simulink model "unit_test"  (R2019a)
settings: Solver=VariableStepAuto  StartTime=0.0  StopTime=inf  RelTol=1e-3
settings Model: Creator=anton  LastModifiedBy=anton

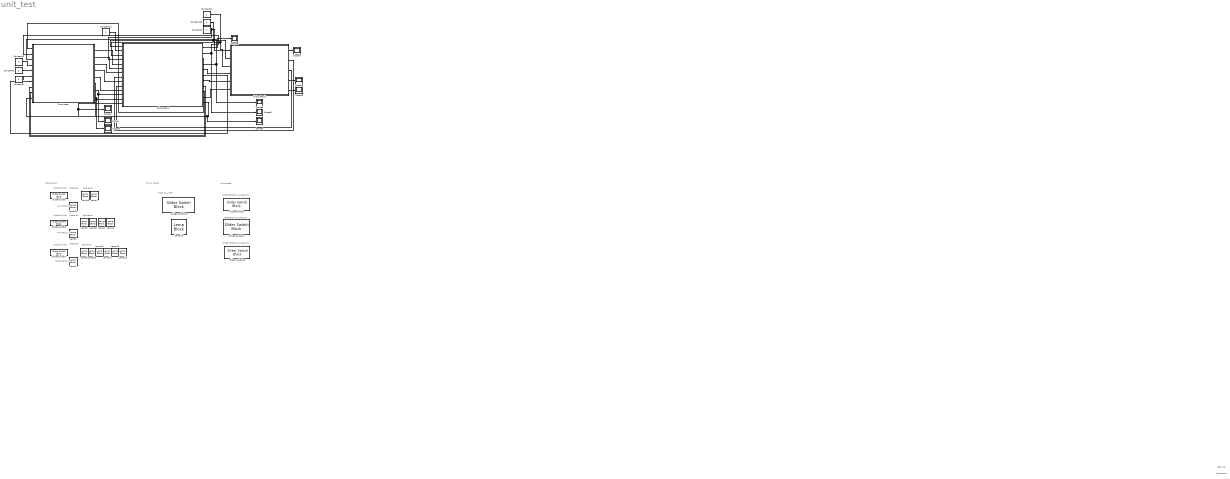
== system unit_test ==
  note: OPERATORE AVAILABILITY
  note: UTENSILE AVAILABILITY
  note: WORKSPACE AVAILABILITY
  note: Workspace
  note: TURN ON / OFF
  note: Pick & Place
  note: Place Pezzo 3
  note: Pick Pezzo 2
  note: Pick Pezzo1
  note: Capienza
  note: Capienza
  note: Capienza
  note: Disponibilità
  note: Scatola3
  note: Scatola2
  note: Scatola1
  note: Warehouse
  note: Operatore
  note: Utensile
  note: Disponibilità
  note: Disponibilità
  Constant{1..4,10..12} (7 alike) : Constant
  Lamp{1..16} (16 alike) : LampBlock
  Scope{,1..9} (10 alike) : Scope
  Slider Switch{,5,7,9,11..13} (7 alike) : SliderSwitchBlock
      settings: Values={{'Off', 'On'}, [0 1]}
  Subsystem : Subsystem
      mask Display: image('F:\MEGAsync\libri\Master\04_Model_Based\Esame\Model-Based-Master\Pick&Place\Immagini\000228601_FR_scatola-cartone-avana-imballi.jpg');
  Subsystem1 : Subsystem
      mask Display: image('967_z_pick_and_place.210.jpg');
  Subsystem2 : Subsystem
      mask Display: image('F:\MEGAsync\libri\Master\04_Model_Based\Esame\Model-Based-Master\Pick&Place\Immagini\download.jpg');
  wires:
  Constant2/1 -> Subsystem2/1(In1), Subsystem1/4(In4)
  Constant12/1 -> Subsystem1/1(In1), Subsystem2/2(In2)
  Constant11/1 -> Subsystem2/3(In3), Subsystem1/3(In3)
  Constant1/1 -> Subsystem/4(In4)
  Constant3/1 -> Subsystem/5(In5)
  Constant4/1 -> Subsystem/6(In6)
  Subsystem2/1(Out1) -> Scope7/1
  Subsystem2/4(Out4) -> Scope8/1
  Subsystem2/5(Out5) -> Scope9/1
  Subsystem/7(Out7) -> Scope/1, Subsystem1/12(In12)
  Subsystem/6(Out6) -> Subsystem1/14(In14), Scope1/1
  Subsystem/8(Out8) -> Scope2/1, Subsystem1/13(In13)
  Subsystem1/4(Out4) -> Scope5/1, Subsystem/3(In3)
  Subsystem1/2(Out2) -> Scope3/1, Subsystem/2(In2)
  Subsystem1/11(Out11) -> Subsystem/10(In10), Scope4/1
  Constant10/1 -> Subsystem1/2(In2)
  Subsystem/1(Out1) -> Subsystem1/5(In5)
  Subsystem/2(Out2) -> Subsystem1/6(In6)
  Subsystem/3(Out3) -> Subsystem1/7(In7)
  Subsystem2/2(Out2) -> Subsystem1/8(In8)
  Subsystem/4(Out4) -> Subsystem1/9(In9)
  Subsystem2/3(Out3) -> Subsystem1/10(In10)
  Subsystem/5(Out5) -> Subsystem1/11(In11)
  Subsystem1/1(Out1) -> Scope6/1
  Subsystem1/3(Out3) -> Subsystem/1(In1)
  Subsystem1/5(Out5) -> Subsystem2/4(In4)
  Subsystem1/6(Out6) -> Subsystem/7(In7)
  Subsystem1/7(Out7) -> Subsystem2/5(In5)
  Subsystem1/8(Out8) -> Subsystem/8(In8)
  Subsystem1/9(Out9) -> Subsystem/9(In9)
  Subsystem1/10(Out10) -> Subsystem2/6(In6)

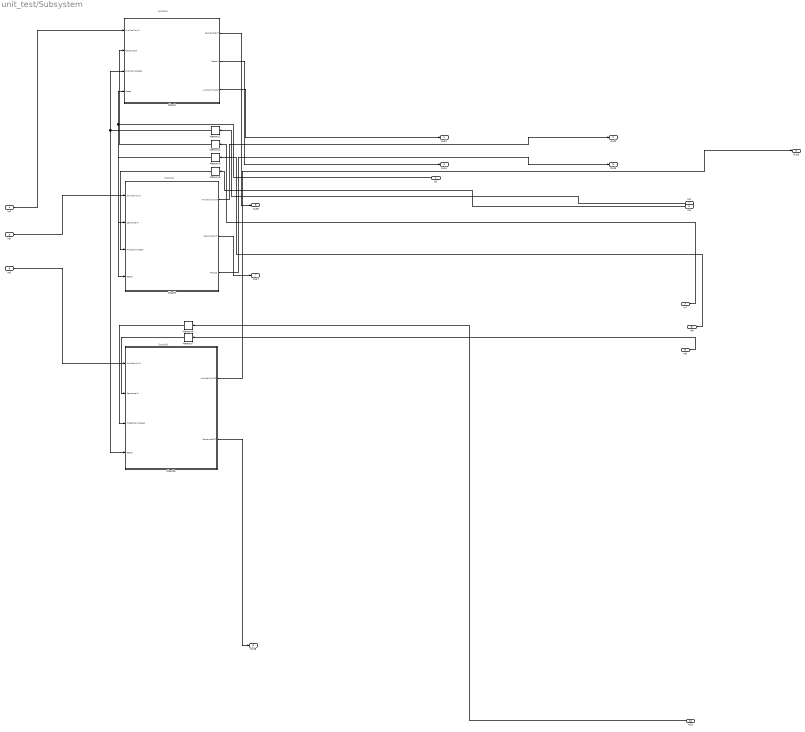
== system unit_test/Subsystem ==
  note: Scatola3
  note: Scatola1
  note: Scatola2
  In1 : Inport
  In2 : Inport  Port=2
  In3 : Inport  Port=3
  In4 : Inport  Port=4
  In5 : Inport  Port=5
  In6 : Inport  Port=6
  In7 : Inport  Port=7
  In8 : Inport  Port=8
  In9 : Inport  Port=9
  In10 : Inport  Port=10
  Chart10 : Stateflow chart  BlockKeywords=__PRM__SERIALIZED__DATA__:Stateflow Chart,Stateflow Diagram  TreatAsAtomicUnit=on
  Chart4 : Stateflow chart  BlockKeywords=__PRM__SERIALIZED__DATA__:Stateflow Chart,Stateflow Diagram  TreatAsAtomicUnit=on
  Chart9 : Stateflow chart  BlockKeywords=__PRM__SERIALIZED__DATA__:Stateflow Chart,Stateflow Diagram  TreatAsAtomicUnit=on
  Memory{1..2,4..7} (6 alike) : Memory
  Out1 : Outport
  Out2 : Outport  Port=2
  Out3 : Outport  Port=3
  Out4 : Outport  Port=4
  Out5 : Outport  Port=5
  Out6 : Outport  Port=6
  Out7 : Outport  Port=7
  Out8 : Outport  Port=8
  wires:
  In10/1 -> Memory6/1
  Memory5/1 -> Chart9/3(Pick2Completed)
  In2/1 -> Memory2/1
  Memory7/1 -> Chart10/2(CapienzaIN)
  Memory1/1 -> Chart4/2(CapienzaIN)
  Memory4/1 -> Chart9/2(CapienzaIN)
  In1/1 -> Chart4/4(Reset), Chart9/4(Reset)
  Chart9/3(Pezzo2) -> Out5/1
  Memory2/1 -> Chart10/4(Reset), Chart4/3(Pick1Completed)
  In6/1 -> Chart10/1(AvailabilityIN)
  Memory6/1 -> Chart10/3(Place3Completed)
  In3/1 -> Memory5/1
  In4/1 -> Chart4/1(AvailabilityIN)
  In5/1 -> Chart9/1(AvailabilityIN)
  In7/1 -> Memory1/1
  Chart10/1(AvailabilityOUT) -> Out3/1
  Chart4/2(Pezzo1) -> Out4/1
  In8/1 -> Memory4/1
  Chart9/1(AvailabilityOUT) -> Out2/1
  In9/1 -> Memory7/1
  Chart9/2(CapienzaOUT) -> Out7/1
  Chart4/1(CapienzaOUT) -> Out6/1
  Chart4/3(AvailabilityOUT) -> Out1/1
  Chart10/2(CapienzaOUT) -> Out8/1

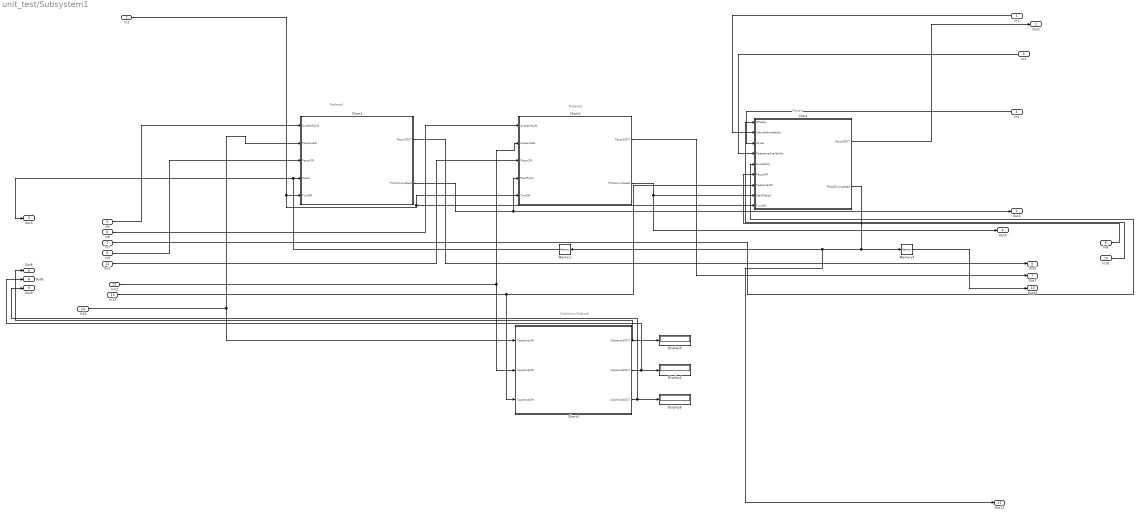
== system unit_test/Subsystem1 ==
  note: Preleva1
  note: Preleva2
  note: Place3
  note: SostituisciScatola
  In1 : Inport
  In2 : Inport  Port=2
  In3 : Inport  Port=3
  In4 : Inport  Port=4
  In5 : Inport  Port=5
  In6 : Inport  Port=6
  In7 : Inport  Port=7
  In8 : Inport  Port=8
  In9 : Inport  Port=9
  In10 : Inport  Port=10
  In11 : Inport  Port=11
  In12 : Inport  Port=12
  In13 : Inport  Port=13
  In14 : Inport  Port=14
  Chart : Stateflow chart  BlockKeywords=__PRM__SERIALIZED__DATA__:Stateflow Chart,Stateflow Diagram  TreatAsAtomicUnit=on
  Chart1 : Stateflow chart  BlockKeywords=__PRM__SERIALIZED__DATA__:Stateflow Chart,Stateflow Diagram  TreatAsAtomicUnit=on
  Chart2 : Stateflow chart  BlockKeywords=__PRM__SERIALIZED__DATA__:Stateflow Chart,Stateflow Diagram  TreatAsAtomicUnit=on
  Chart3 : Stateflow chart  BlockKeywords=__PRM__SERIALIZED__DATA__:Stateflow Chart,Stateflow Diagram  TreatAsAtomicUnit=on
  Display3 : Display
  Display4 : Display
  Display5 : Display
  Memory : Memory
  Memory3 : Memory
  Out1 : Outport
  Out2 : Outport  Port=2
  Out3 : Outport  Port=3
  Out4 : Outport  Port=4
  Out5 : Outport  Port=5
  Out6 : Outport  Port=6
  Out7 : Outport  Port=7
  Out8 : Outport  Port=8
  Out9 : Outport  Port=9
  Out10 : Outport  Port=10
  Out11 : Outport  Port=11
  wires:
  In2/1 -> Chart/9(TurnON), Chart2/5(TurnON), Chart1/5(TurnON)
  Chart/2(Place3Completed) -> Out11/1, Memory/1, Memory3/1
  In13/1 -> Chart3/3(Capienza3IN), Chart/7(Capienza3IN)
  In9/1 -> Chart1/3(Pezzo1IN)
  In12/1 -> Chart3/2(Capienza2IN), Chart2/2(CapienzaIN)
  In14/1 -> Chart1/2(CapienzaIN), Chart3/1(Capienza1IN)
  Memory/1 -> Out3/1, Chart1/4(Reset)
  Chart1/2(Pick1Completed) -> Out2/1, Chart2/4(StartPick2)
  In7/1 -> Chart/5(Availability)
  Chart3/1(Capienza1OUT) -> Out6/1, Display3/1
  In1/1 -> Chart/2(UtensileAvailability)
  Chart2/2(Pick2Completed) -> Out4/1, Chart/8(StartPlace3)
  Chart3/2(Capienza2OUT) -> Out8/1, Display4/1
  Chart3/3(Capienza3OUT) -> Out9/1, Display5/1
  In3/1 -> Chart/4(OperatoreAvailability)
  In6/1 -> Chart2/1(AvailabilityIN)
  Chart2/1(Pezzo2OUT) -> Out7/1
  In4/1 -> Chart/3(IsFree)
  In10/1 -> Chart/1(IsReady)
  Memory3/1 -> Out10/1
  Chart/1(Pezzo3OUT) -> Out1/1
  In8/1 -> Chart/6(Pezzo3IN)
  In11/1 -> Chart2/3(Pezzo2IN)
  In5/1 -> Chart1/1(AvailabilityIN)
  Chart1/1(Pezzo1OUT) -> Out5/1

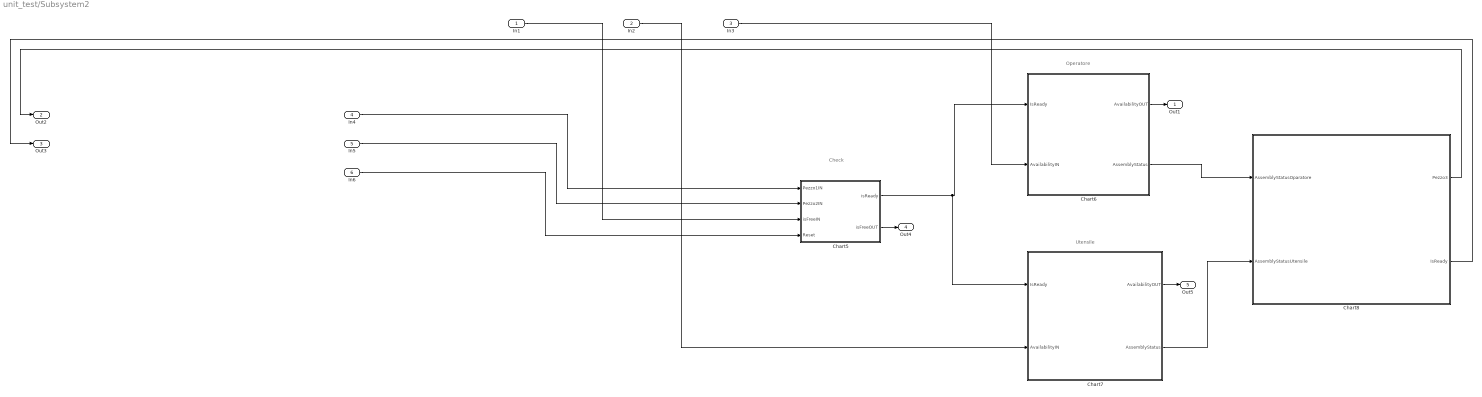
== system unit_test/Subsystem2 ==
  note: Check
  note: Operatore
  note: Utensile
  In1 : Inport
  In2 : Inport  Port=2
  In3 : Inport  Port=3
  In4 : Inport  Port=4
  In5 : Inport  Port=5
  In6 : Inport  Port=6
  Chart5 : Stateflow chart  BlockKeywords=__PRM__SERIALIZED__DATA__:Stateflow Chart,Stateflow Diagram  TreatAsAtomicUnit=on
  Chart6 : Stateflow chart  BlockKeywords=__PRM__SERIALIZED__DATA__:Stateflow Chart,Stateflow Diagram  TreatAsAtomicUnit=on
  Chart7 : Stateflow chart  BlockKeywords=__PRM__SERIALIZED__DATA__:Stateflow Chart,Stateflow Diagram  TreatAsAtomicUnit=on
  Chart8 : Stateflow chart  BlockKeywords=__PRM__SERIALIZED__DATA__:Stateflow Chart,Stateflow Diagram  TreatAsAtomicUnit=on
  Out1 : Outport
  Out2 : Outport  Port=2
  Out3 : Outport  Port=3
  Out4 : Outport  Port=4
  Out5 : Outport  Port=5
  wires:
  In1/1 -> Chart5/3(isFreeIN)
  Chart5/1(isReady) -> Chart7/1(IsReady), Chart6/1(IsReady)
  Chart5/2(isFreeOUT) -> Out4/1
  In3/1 -> Chart6/2(AvailabilityIN)
  Chart7/1(AvailabilityOUT) -> Out5/1
  Chart6/2(AssemblyStatus) -> Chart8/1(AssemblyStatusOparatore)
  Chart7/2(AssemblyStatus) -> Chart8/2(AssemblyStatusUtensile)
  In4/1 -> Chart5/1(Pezzo1IN)
  In2/1 -> Chart7/2(AvailabilityIN)
  In5/1 -> Chart5/2(Pezzo2IN)
  Chart8/2(IsReady) -> Out3/1
  Chart8/1(Pezzo3) -> Out2/1
  In6/1 -> Chart5/4(Reset)
  Chart6/1(AvailabilityOUT) -> Out1/1

== stateflow chart unit_test/Subsystem1/Chart1 ==
  state Idle
    Pezzo1OUT=0;
    Pick1Completed=0;
  state Waiting
    Pezzo1OUT=0;
    Pick1Completed=0;
  state Active
  state Working
  state Place
    during:
    Pezzo1OUT=1;
    Pick1Completed = 1;
  state Pick
    pause(0.1);
  (default) -> Idle
  Place -> Idle [order 1] : [TurnON==0]
  Idle -> Active : [TurnON==1]
  Waiting -> Idle [order 2] : [TurnON==0]
  Pick -> Idle [order 2] : [TurnON==0]
  Working -> Idle [order 2] : [TurnON==0]
  Active -> Working
  Place -> Waiting [order 2] : [after(1,sec)]
  Waiting -> Working [order 1] : [Reset==1]
  Working -> Pick [order 1] : [AvailabilityIN==1 && CapienzaIN>0 && Pezzo1IN==1]
  Pick -> Place [order 1] : [after(5,sec)]
  data: AvailabilityIN input; CapienzaIN input; Pezzo1IN input; Pezzo1OUT output; Pick1Completed output; Reset input; TurnON input

== stateflow chart unit_test/Subsystem1/Chart2 ==
  state Idle
    Pezzo2OUT=0;
    Pick2Completed=0;
  state Waiting
    Pezzo2OUT=0;
    Pick2Completed=0;
  state Active
  state Working
  state Place
    during:
    Pezzo2OUT=1;
    Pick2Completed = 1;
    pause(0.1);
  state Pick
    pause(0.1);
  (default) -> Idle
  Idle -> Active : [TurnON==1]
  Place -> Idle [order 2] : [TurnON==0]
  Waiting -> Idle [order 2] : [TurnON==0]
  Pick -> Idle [order 2] : [TurnON==0]
  Working -> Idle [order 2] : [TurnON==0]
  Active -> Waiting
  Waiting -> Working [order 1] : [StartPick2==1]
  Place -> Waiting [order 1] : [after(1,sec)]
  Working -> Pick [order 1] : [AvailabilityIN==1 && CapienzaIN>0 && Pezzo2IN==1]
  Pick -> Place [order 1] : [after(5,sec)]
  data: AvailabilityIN input; CapienzaIN input; Pezzo2IN input; Pezzo2OUT output; StartPick2 input; Pick2Completed output; TurnON input

== stateflow chart unit_test/Subsystem1/Chart ==
  state Idle
    Pezzo3OUT=0;
    Place3Completed=0;
  state Waiting
    Pezzo3OUT=0;
    Place3Completed=0;
  state Active1
  state Working
  state Place
    during:
    Pezzo3OUT=1;
    Place3Completed = 1;
    pause(0.1);
  state Pick
    pause(0.1);
  (default) -> Idle
  Idle -> Active1 : [TurnON==1]
  Place -> Idle [order 2] : [TurnON==0]
  Waiting -> Idle [order 2] : [TurnON==0]
  Pick -> Idle [order 2] : [TurnON==0]
  Working -> Idle [order 2] : [TurnON==0]
  Active1 -> Waiting
  Waiting -> Working [order 1] : [StartPlace3==1]
  Place -> Waiting [order 1] : [after(1,sec)]
  Working -> Pick [order 1] : [IsReady==1 && Availability==1 && Pezzo3IN==1 && Capienza3IN<6 && IsFree==1 && (UtensileAvailability==1 || OperatoreAvailability==1)]
  Pick -> Place [order 1] : [after(5,sec)]
  data: IsReady input; UtensileAvailability input; IsFree input; OperatoreAvailability input; Availability input; Pezzo3IN input; Capienza3IN input; StartPlace3 input; Pezzo3OUT output; Place3Completed output; TurnON input

== stateflow chart unit_test/Subsystem1/Chart3 ==
  state Idle
    Capienza1OUT=0;
    Capienza2OUT=0;
    Capienza3OUT=0;
  state Scatola1Expired
    Capienza1OUT=1;
  state Scatola2Expired
    Capienza2OUT=1;
  state Scatola3Expired
    Capienza3OUT=1;
  (default) -> Idle
  Idle -> Scatola1Expired [order 1] : [Capienza1IN<=0]
  Idle -> Scatola3Expired [order 3] : [Capienza3IN>=6]
  Scatola3Expired -> Idle
  Scatola1Expired -> Idle
  Scatola2Expired -> Idle
  Idle -> Scatola2Expired [order 2] : [Capienza2IN<=0]
  data: Capienza1IN input; Capienza2IN input; Capienza3IN input; Capienza1OUT output; Capienza2OUT output; Capienza3OUT output

== stateflow chart unit_test/Subsystem/Chart4 ==
  state Idle
    CapienzaOUT=2;
    AvailabilityOUT=AvailabilityIN;
    pause(0.1);
  state Capienza2
    CapienzaOUT=2;
    Pezzo1=1;
    AvailabilityOUT=AvailabilityIN;
    pause(0.1);
  state Waiting
    CapienzaOUT=1;
  state Capienza1
    CapienzaOUT=1;
    Pezzo1=1;
    AvailabilityOUT=AvailabilityIN;
    pause(0.1);
  state Waiting1
    CapienzaOUT=0;
  state Capienza0
    CapienzaOUT=0;
    Pezzo1=0;
    AvailabilityOUT=AvailabilityIN;
    pause(0.1);
  (default) -> Idle
  Capienza0 -> Idle : [CapienzaIN==1]
  Idle -> Capienza2
  Capienza2 -> Waiting : [Pick1Completed==1]
  Waiting -> Capienza1 : [Reset==1]
  Capienza1 -> Waiting1 : [Pick1Completed==1]
  Waiting1 -> Capienza0 : [Reset==1]
  data: AvailabilityIN input; CapienzaOUT output; Pezzo1 output; AvailabilityOUT output; CapienzaIN input; Pick1Completed input; Reset input

== stateflow chart unit_test/Subsystem2/Chart5 ==
  state Idle
    isReady = 0;
  state Pezzo1Available
  state Pezzo2Available
  state Check
    isReady = 1;
    isFreeOUT = 1;
  (default) -> Idle
  Check -> Idle : [Reset==1]
  Idle -> Pezzo1Available : [Pezzo1IN==1]
  Pezzo1Available -> Pezzo2Available : [Pezzo2IN==1]
  Pezzo2Available -> Check : [isFreeIN == 1]
  data: isReady output; isFreeOUT output; Pezzo1IN input; Pezzo2IN input; isFreeIN input; Reset input

== stateflow chart unit_test/Subsystem2/Chart6 ==
  state CheckDisponibility
    if IsReady == 1 && AvailabilityIN == 1
    AvailabilityOUT = AvailabilityIN;
    AssemblyStatus = 1;
    end
  (default) -> CheckDisponibility
  data: AvailabilityOUT output; AssemblyStatus output; IsReady input; AvailabilityIN input

== stateflow chart unit_test/Subsystem2/Chart7 ==
  state CheckDisponibility
    if IsReady == 1 && AvailabilityIN == 1
    AvailabilityOUT = AvailabilityIN;
    AssemblyStatus = 1;
    end
  (default) -> CheckDisponibility
  data: IsReady input; AvailabilityIN input; AvailabilityOUT output; AssemblyStatus output

== stateflow chart unit_test/Subsystem2/Chart8 ==
  state Montage
    if AssemblyStatusOparatore == 1 || AssemblyStatusUtensile == 1
    IsReady = 1;
    Pezzo3 = 1;
    end
  (default) -> Montage
  data: Pezzo3 output; IsReady output; AssemblyStatusOparatore input; AssemblyStatusUtensile input

== stateflow chart unit_test/Subsystem/Chart9 ==
  state Idle
    CapienzaOUT=4;
    AvailabilityOUT=AvailabilityIN;
    pause(0.1);
  state Capienza4
    CapienzaOUT=4;
    Pezzo2=1;
    AvailabilityOUT=AvailabilityIN;
    pause(0.1);
  state Waiting3
    CapienzaOUT=3;
  state Capienza3
    CapienzaOUT=3;
    Pezzo2=1;
    AvailabilityOUT=AvailabilityIN;
    pause(0.1);
  state Waiting2
    CapienzaOUT=2;
  state Capienza2
    CapienzaOUT=2;
    Pezzo2=1;
    AvailabilityOUT=AvailabilityIN;
    pause(0.1);
  state Waiting
    CapienzaOUT=1;
  state Capienza1
    CapienzaOUT=1;
    Pezzo2=1;
    AvailabilityOUT=AvailabilityIN;
    pause(0.1);
  state Waiting1
    CapienzaOUT=0;
  state Capienza0
    CapienzaOUT=0;
    Pezzo2=0;
    AvailabilityOUT=AvailabilityIN;
    pause(0.1);
  (default) -> Idle
  Capienza0 -> Idle : [CapienzaIN==1]
  Idle -> Capienza4
  Capienza4 -> Waiting3 : [Pick2Completed==1]
  Waiting3 -> Capienza3 : [Reset==1]
  Capienza3 -> Waiting2 : [Pick2Completed==1]
  Waiting2 -> Capienza2 : [Reset==1]
  Capienza2 -> Waiting : [Pick2Completed==1]
  Waiting -> Capienza1 : [Reset==1]
  Capienza1 -> Waiting1 : [Pick2Completed==1]
  Waiting1 -> Capienza0 : [Reset==1]
  data: AvailabilityIN input; CapienzaIN input; Pick2Completed input; Reset input; AvailabilityOUT output; CapienzaOUT output; Pezzo2 output

== stateflow chart unit_test/Subsystem/Chart10 ==
  state Idle
    CapienzaOUT=0;
    AvailabilityOUT=AvailabilityIN;
    pause(0.1);
  state Capienza6
    CapienzaOUT=0;
    AvailabilityOUT=AvailabilityIN;
    pause(0.1);
  state Capienza5
    CapienzaOUT=1;
    AvailabilityOUT=AvailabilityIN;
    pause(0.1);
  state Waiting4
  state Capienza4
    CapienzaOUT=2;
    AvailabilityOUT=AvailabilityIN;
    pause(0.1);
  state Waiting3
  state Capienza3
    CapienzaOUT=3;
    AvailabilityOUT=AvailabilityIN;
    pause(0.1);
  state Waiting2
  state Capienza2
    CapienzaOUT=4;
    AvailabilityOUT=AvailabilityIN;
    pause(0.1);
  state Waiting
  state Capienza1
    CapienzaOUT=5;
    AvailabilityOUT=AvailabilityIN;
    pause(0.1);
  state Waiting1
  state Capienza0
    CapienzaOUT=6;
    AvailabilityOUT=AvailabilityIN;
    pause(0.1);
  (default) -> Idle
  Capienza0 -> Idle : [CapienzaIN==1]
  Idle -> Capienza6
  Capienza6 -> Capienza5 : [Place3Completed==1]
  Capienza5 -> Waiting4 : [Reset==1]
  Waiting4 -> Capienza4 : [Place3Completed==1]
  Capienza4 -> Waiting3 : [Reset==1]
  Waiting3 -> Capienza3 : [Place3Completed==1]
  Capienza3 -> Waiting2 : [Reset==1]
  Waiting2 -> Capienza2 : [Place3Completed==1]
  Capienza2 -> Waiting : [Reset==1]
  Waiting -> Capienza1 : [Place3Completed==1]
  Capienza1 -> Waiting1 : [Reset==1]
  Waiting1 -> Capienza0 : [Place3Completed==1]
  data: AvailabilityIN input; CapienzaIN input; Place3Completed input; Reset input; AvailabilityOUT output; CapienzaOUT output
